simulink library "EnergyMeter"  (Simulink 8.2)
settings: Solver=ode45  StartTime=0.0  StopTime=10.0  RelTol=1e-3
libraries: carnot x1
settings Model: Creator=lena.frank  LastModifiedBy=drhf

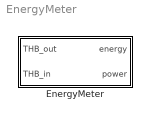
== system EnergyMeter ==
  EnergyMeter : Subsystem  mask(energy meter){}
      mask help: Calculates the power and energy of a fluid flow between inlet and outlet of components.
      mask Help: web(fullfile(path_carnot('help'),'EnergyMeter.html'),'-helpbrowser')

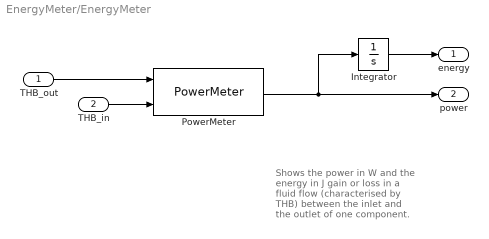
== system EnergyMeter/EnergyMeter ==
  note: Shows the power in W and the energy in J gain or loss
      | in a fluid flow (characterised by THB) between the
      | inlet and the outlet of one component.
  THB_out : Inport
  THB_in : Inport  Port=2
  Integrator : Integrator  UpperSaturationLimit=1  LowerSaturationLimit=0
  PowerMeter : carnot/Control/PowerMeter
  energy : Outport
  power : Outport  Port=2
  wires:
  PowerMeter/1 -> Integrator/1, power/1
  THB_in/1 -> PowerMeter/2
  Integrator/1 -> energy/1
  THB_out/1 -> PowerMeter/1
